simulink subsystem "EngineCustom_refsub"  (R2022a)
settings: Solver=VariableStepAuto  StartTime=0.0  StopTime=10.0  RelTol=1e-3
undefined symbols (not defined in the file): engine
libraries: fl_lib x13, nesl_utility x3, sdl_lib x1
settings Model: Creator=isaacito  LastModifiedBy=isaacito
settings SolverCC: AlgebraicLoopSolver=TrustRegion
settings DebuggingCC: UnconnectedInputMsg=warning  UnconnectedOutputMsg=warning  UnconnectedLineMsg=warning  SFMachineParentedDataDiag=warning
settings RTWCC: DLArmComputeVersion=19.05

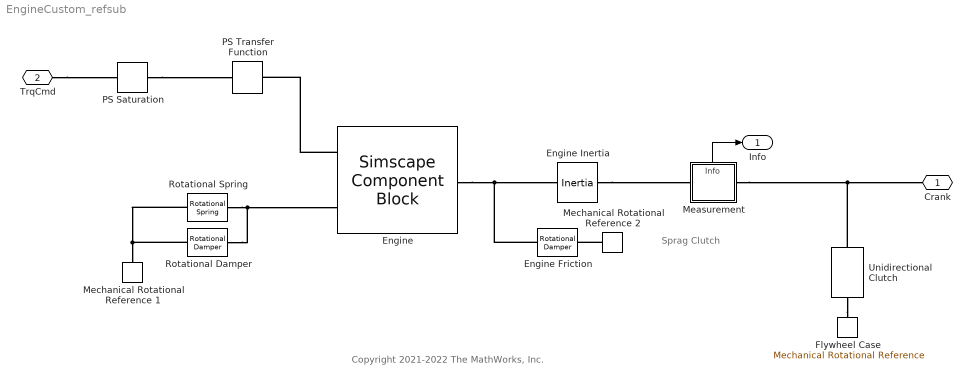
== system EngineCustom_refsub ==
  note: Copyright 2021-2022 The MathWorks, Inc.
  note: Sprag Clutch
  Engine : SimscapeComponentBlock  SourceFile=EngineCustom  ComponentPath=EngineCustom  ComponentVariants="[\"EngineCustom\"]"  ComponentVariantNames="[\"EngineCustom\"]"  ClassName=EngineCustom  SchemaVersion=1  PeakTorque=engine.trqMax_Nm N*m  PeakTorqueSpeed=engine.trqMaxSpd_rpm rpm  PeakPower=engine.powerMax_kW kW  MaxSpeed=engine.maxSpd_rpm rpm  StallSpeed=engine.stallSpd_rpm rpm  SmoothingWidth=engine.smoothing_rpm rpm  w_specify=on  w_priority=High  w=initial.engine_speed_rpm rpm  w_nominal_specify=off  w_nominal_unit=rad/s  w_nominal_value=1  trq_specify=off  trq_priority=None  trq=0 N*m  trq_nominal_specify=off  trq_nominal_unit=N*m  trq_nominal_value=1
      settings: CopyFcn=simscape.engine.sli.internal.componentblockcallback(gcbh,'COPY')  PreCopyFcn=simscape.engine.sli.internal.componentblockcallback(gcbh,'PRECOPY')  PreDeleteFcn=simscape.engine.sli.internal.componentblockcallback(gcbh,'PREDELETE')  InternalSimscapePortConfiguration="{\"Bottom\":[],\"Left\":[{\"id\":\"TrqCmdIn\",\"label\":\"TrqCmd\",\"type\":\"input\"},{\"id\":\"B\",\"label\":\"B\",\"type\":\"foundation.mechanical.rotational.rotational\"}],\"Right\":[{\"id\":\"F\",\"label\":\"F\",\"type\":\"foundation.mechanical.rotational.rotational\"}],\"Top\":[]}"
      mask Type: Abstract Engine Model
  Engine Friction : fl_lib/Mechanical/Rotational Elements/Rotational Damper  D=engine.damping_Nm_per_rpm m*N/rpm  w_specify=off  w_priority=None  w=0 rad/s  w_nominal_specify=off  w_nominal_unit=rad/s  w_nominal_value=1  t_specify=off  t_priority=None  t=0 N*m  t_nominal_specify=off  t_nominal_unit=N*m  t_nominal_value=1
      settings: SourceProductBaseCode=PW,SS,VE
  Engine Inertia : fl_lib/Mechanical/Rotational Elements/Inertia  inertia=engine.inertia_kg_m2 kg*m^2  num_ports=foundation.enum.numPorts2.two  w_specify=on  w_priority=None  w=initial.engine_speed_rpm rpm  w_nominal_specify=off  w_nominal_unit=rad/s  w_nominal_value=1  t_specify=off  t_priority=None  t=0 N*m  t_nominal_specify=off  t_nominal_unit=N*m  t_nominal_value=1
      settings: SourceProductBaseCode=PW,SS,VE  InternalSimscapePortConfiguration="{\"Bottom\":[],\"Left\":[{\"id\":\"I\",\"label\":\"\",\"type\":\"foundation.mechanical.rotational.rotational\"}],\"Right\":[{\"id\":\"J\",\"label\":\"\",\"type\":\"foundation.mechanical.rotational.rotational\"}],\"Top\":[]}"
      settings: AttributesFormatString=|
      | %<inertia> (%<inertia_unit>)
      | %<w> (%<w_unit>)
      | Priority: %<w_priority>
  Flywheel Case : fl_lib/Mechanical/Rotational Elements/Mechanical Rotational Reference
      settings: SourceProductBaseCode=PW,SS,VE
  Measurement : Subsystem
      settings: PortSchema="{\"entries\":[{\"content\":{\"sides\":[{\"content\":{\"connectorIds\":[\"LConn1\"]},\"type\":\"ConnectorPlacement.EquallySpacedRectSide\",\"uuid\":\"07c2ae95-e870-4b8d-a90d-f6f29bd91438\"},{\"content\":{\"connectorIds\":[\"RConn1\"],\"side\":\"RIGHT\"},\"type\":\"ConnectorPlacement.EquallySpacedRectSide\",\"uuid\":\"a6bad6b4-02de-43bd-83c0-90c7caa8debd\"},{\"content\":{\"connectorIds\":[\"Out1\"],\"side\":\"TOP\"},\"type\":\"ConnectorPlacement.EquallySpacedRectSide\",\"uuid\":\"e2b5c796-e9a6-4d01-87a6-78788a72fccc\"}]},\"type\":\"ConnectorPlacement.EquallySpacedConnector\",\"uuid\":\"494e0008-7a6b-45d1-a26f-72f06cc564cf\"}],\"packageUris\":[\"http://schema.mathworks.com/mf0/Connector/R2020b\"],\"version\":\"1.0\"}"
  Mechanical Rotational Reference 1 : fl_lib/Mechanical/Rotational Elements/Mechanical Rotational Reference
      settings: SourceProductBaseCode=PW,SS,VE
  Mechanical Rotational Reference 2 : fl_lib/Mechanical/Rotational Elements/Mechanical Rotational Reference
      settings: SourceProductBaseCode=PW,SS,VE
  PS Saturation : fl_lib/Physical Signals/Nonlinear Operators/PS Saturation  upper_limit=engine.trqMax_Nm N*m  lower_limit=0 N*m
      settings: AttributesFormatString=%<upper_limit> (%<upper_limit_unit>)  SourceProductBaseCode=PW,SS,VE
  PS Transfer Function : fl_lib/Physical Signals/Linear Operators/PS Transfer Function  transfer_function_type=foundation.enum.transfer_function_type.lag  T=engine.lag_s s  T1=2 s  T2=1 s  y0=initial.engine_torque_Nm N*m
      settings: SourceProductBaseCode=PW,SS,VE  InternalSimscapePortConfiguration="{\"Bottom\":[],\"Left\":[{\"id\":\"U\",\"label\":\"\",\"type\":\"input\"}],\"Right\":[{\"id\":\"Y\",\"label\":\"\",\"type\":\"output\"}],\"Top\":[]}"
      settings: AttributesFormatString=|
      | %<T> [%<T_unit>]
      | Initial: %<y0> [%<y0_unit>]
  Rotational Damper : fl_lib/Mechanical/Rotational Elements/Rotational Damper  D=engine.dampSpringFriction_Nm_per_rpm N*m/rpm  w_specify=off  w_priority=None  w=0 rad/s  w_nominal_specify=off  w_nominal_unit=rad/s  w_nominal_value=1  t_specify=off  t_priority=None  t=0 N*m  t_nominal_specify=off  t_nominal_unit=N*m  t_nominal_value=1
      settings: SourceProductBaseCode=PW,SS,VE
  Rotational Spring : fl_lib/Mechanical/Rotational Elements/Rotational Spring  spr_rate=engine.dampSpringStiffness_Nm_per_rad N*m/rad  w_specify=off  w_priority=None  w=0 rad/s  w_nominal_specify=off  w_nominal_unit=rad/s  w_nominal_value=1  t_specify=off  t_priority=None  t=0 N*m  t_nominal_specify=off  t_nominal_unit=N*m  t_nominal_value=1  phi_specify=on  phi_priority=Low  phi=0 rad  phi_nominal_specify=off  phi_nominal_unit=rad  phi_nominal_value=1
      settings: AttributesFormatString=Deformation priority: %<phi_priority>  SourceProductBaseCode=PW,SS,VE
  Unidirectional Clutch : sdl_lib/Clutches/Unidirectional Clutch  transmission_direction=2  initial_state_locked=sdl.enum.initial_lock.unlocked
      settings: AttributesFormatString=%<initial_state_locked>  SourceProductBaseCode=LD  InternalSimscapePortConfiguration="{\"Bottom\":[],\"Left\":[{\"id\":\"H\",\"label\":\"H\",\"type\":\"foundation.mechanical.rotational.rotational\"}],\"Right\":[{\"id\":\"R\",\"label\":\"R\",\"type\":\"foundation.mechanical.rotational.rotational\"}],\"Top\":[]}"
  Crank : PMIOPort  Side=Left
  TrqCmd : PMIOPort  Port=2  Side=Right
  Info : Outport
  wires:
  Measurement/1(Info) -> Info/1
  connections:
  Rotational Spring/RConn1 -- Rotational Damper/RConn1 -- Engine/LConn2
  Rotational Spring/LConn1 -- Rotational Damper/LConn1 -- Mechanical Rotational Reference 1/LConn1
  Unidirectional Clutch/LConn1 -- Measurement/RConn1 -- Crank/RConn1
  Engine Friction/LConn1 -- Engine Inertia/RConn1 -- Engine/RConn1
  Unidirectional Clutch/RConn1 -- Flywheel Case/LConn1
  Engine Inertia/LConn1 -- Measurement/LConn1
  Engine/LConn1 -- PS Transfer Function/RConn1
  Mechanical Rotational Reference 2/LConn1 -- Engine Friction/RConn1
  TrqCmd/RConn1 -- PS Saturation/LConn1
  PS Saturation/RConn1 -- PS Transfer Function/LConn1

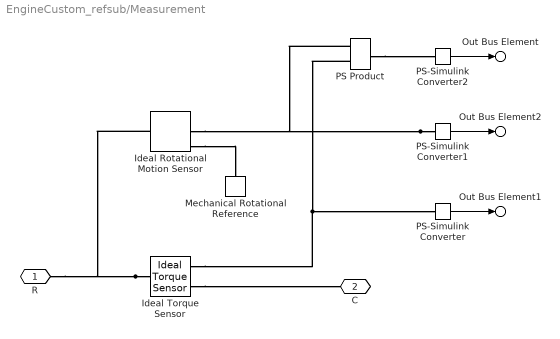
== system EngineCustom_refsub/Measurement ==
  Ideal Rotational Motion Sensor : fl_lib/Mechanical/Mechanical Sensors/Ideal Rotational Motion Sensor  wrap_angle=simscape.enum.onoff.off  offset=0 rad
      settings: SourceProductBaseCode=PW,SS,VE
  Ideal Torque Sensor : fl_lib/Mechanical/Mechanical Sensors/Ideal Torque Sensor
      settings: SourceProductBaseCode=PW,SS,VE
  Mechanical Rotational Reference : fl_lib/Mechanical/Rotational Elements/Mechanical Rotational Reference
      settings: SourceProductBaseCode=PW,SS,VE
  PS Product : fl_lib/Physical Signals/Functions/PS Product
      settings: SourceProductBaseCode=PW,SS,VE
  PS-Simulink Converter : nesl_utility/PS-Simulink Converter  PhysicalDomain=network_engine_domain  SubClassName=ps_output  LeftPortType=input  RightPortType=output  PseudoPeriodic=off  Frequencies=[]  VectorFormat=1-D array  Unit=N*m  AffineConversion=off
      settings: SourceProductBaseCode=SS,PW,VE
  PS-Simulink Converter1 : nesl_utility/PS-Simulink Converter  PhysicalDomain=network_engine_domain  SubClassName=ps_output  LeftPortType=input  RightPortType=output  PseudoPeriodic=off  Frequencies=[]  VectorFormat=1-D array  Unit=rpm  AffineConversion=off
      settings: SourceProductBaseCode=SS,PW,VE
  PS-Simulink Converter2 : nesl_utility/PS-Simulink Converter  PhysicalDomain=network_engine_domain  SubClassName=ps_output  LeftPortType=input  RightPortType=output  PseudoPeriodic=off  Frequencies=[]  VectorFormat=1-D array  Unit=kW  AffineConversion=off
      settings: SourceProductBaseCode=SS,PW,VE
  R : PMIOPort  Side=Left
  C : PMIOPort  Port=2  Side=Right
  Out Bus Element : Outport  PortName=Info  Element=EngPwr
  Out Bus Element1 : Outport  PortName=Info  Element=EngTrq
  Out Bus Element2 : Outport  PortName=Info  Element=EngSpd
  wires:
  PS-Simulink Converter1/1 -> Out Bus Element2/1
  PS-Simulink Converter/1 -> Out Bus Element1/1
  PS-Simulink Converter2/1 -> Out Bus Element/1
  connections:
  PS Product/RConn1 -- PS-Simulink Converter2/LConn1
  Ideal Rotational Motion Sensor/RConn1 -- Mechanical Rotational Reference/LConn1
  Ideal Torque Sensor/LConn1 -- R/RConn1 -- Ideal Rotational Motion Sensor/LConn1
  Ideal Torque Sensor/RConn1 -- C/RConn1
  PS Product/LConn2 -- Ideal Torque Sensor/RConn2 -- PS-Simulink Converter/LConn1
  PS-Simulink Converter1/LConn1 -- Ideal Rotational Motion Sensor/RConn2 -- PS Product/LConn1
